simulink model "Detumbling_project"  (R2022b)
settings: Solver=VariableStepAuto  StartTime=0.0  StopTime=400  RelTol=1e-3
values from neighbouring files (symbols this model uses):
  a = (Rp+Ra)/2    [trial_complete_project.m]    (also in trial_detumbling.m; trial_earth_pointing.m)
  A0 = Ax*Ay*Az    [trial_complete_project.m]    (also in trial_detumbling.m = [0.5391 0.1008 0.8362; -0.3591 0.9255 0.1200; -0.7618 -0.365; trial_earth_pointing.m = [-0.2505 -0.7848 0.5668; 0.7978 0.1644 0.5801; -0.5485 0.597)
  A1 = L1*L2    (= 0.06)    [trial_complete_project.m]    (also in trial_detumbling.m; trial_earth_pointing.m)
  A10 = A1    (= 0.06)    [trial_complete_project.m]    (also in trial_detumbling.m; trial_earth_pointing.m)
  A2 = A1    (= 0.06)    [trial_complete_project.m]    (also in trial_detumbling.m; trial_earth_pointing.m)
  A3 = L1*L3    (= 0.03)    [trial_complete_project.m]    (also in trial_detumbling.m; trial_earth_pointing.m)
  A4 = A3    (= 0.03)    [trial_complete_project.m]    (also in trial_detumbling.m; trial_earth_pointing.m)
  A5 = L2*L3    (= 0.02)    [trial_complete_project.m]    (also in trial_detumbling.m; trial_earth_pointing.m)
  A6 = A5    (= 0.02)    [trial_complete_project.m]    (also in trial_detumbling.m; trial_earth_pointing.m)
  A7 = A1    (= 0.06)    [trial_complete_project.m]    (also in trial_detumbling.m; trial_earth_pointing.m)
  A8 = A1    (= 0.06)    [trial_complete_project.m]    (also in trial_detumbling.m; trial_earth_pointing.m)
  A9 = A1    (= 0.06)    [trial_complete_project.m]    (also in trial_detumbling.m; trial_earth_pointing.m)
  a_s = 149600000    [trial_complete_project.m]    (also in trial_detumbling.m; trial_earth_pointing.m)
  alpha1 = 0.9    [trial_complete_project.m]    (also in trial_detumbling.m; trial_earth_pointing.m)
  alpha2 = 0.1    [trial_complete_project.m]    (also in trial_detumbling.m; trial_earth_pointing.m)
  alphaState_obs = -0.9    [trial_complete_project.m]    (also in trial_detumbling.m; trial_earth_pointing.m)
  an = (11.5*pi)/180    (= 0.200712863979)    [trial_complete_project.m]    (also in trial_detumbling.m; trial_earth_pointing.m)
  d = 0.05/2    (= 0.025)    [trial_complete_project.m]    (also in trial_detumbling.m; trial_earth_pointing.m)
  e = (Ra-Rp)/(Ra+Rp)    [trial_complete_project.m]    (also in trial_detumbling.m; trial_earth_pointing.m)
  e_s = 0.0167086    [trial_complete_project.m]    (also in trial_detumbling.m; trial_earth_pointing.m)
  g_vect = g_vect'.*1e-9    [trial_complete_project.m]    (also in trial_detumbling.m; trial_earth_pointing.m)
  gamma = 30*pi/180    (= 0.523598775598)    [trial_complete_project.m]    (also in trial_detumbling.m; trial_earth_pointing.m)
  h_vect = h_vect'.*1e-9    [trial_complete_project.m]    (also in trial_detumbling.m; trial_earth_pointing.m)
  i = 0*pi/180    (= 0)    [trial_complete_project.m]    (also in trial_detumbling.m; trial_earth_pointing.m)
  I_x = 0.059029338    [trial_complete_project.m]    (also in trial_detumbling.m; trial_earth_pointing.m = 0.093296)
  I_y = 0.116709338    [trial_complete_project.m]    (also in trial_detumbling.m; trial_earth_pointing.m = 0.161261916)
  I_z = 0.149968    [trial_complete_project.m]    (also in trial_detumbling.m; trial_earth_pointing.m = 0.160253916)
  kdx = kd*(I_x/I)    (= 1.44987726319)    [trial_complete_project.m]    (also in trial_detumbling.m; trial_earth_pointing.m = 2.6989394073)
  kdy = kd*(I_y/I)    (= 2.86661211697)    [trial_complete_project.m]    (also in trial_detumbling.m; trial_earth_pointing.m = 4.66511040119)
  kdz = kd*(I_z/I)    (= 3.68351061984)    [trial_complete_project.m]    (also in trial_detumbling.m; trial_earth_pointing.m = 4.63595019151)
  kState_obs = 0.9    [trial_complete_project.m]    (also in trial_detumbling.m; trial_earth_pointing.m)
  L = 0.3/2    (= 0.15)    [trial_complete_project.m]    (also in trial_detumbling.m; trial_earth_pointing.m)
  m = [0.01 0.05 0.01]    [trial_complete_project.m]    (also in trial_detumbling.m; trial_earth_pointing.m)
  MIB = 5*1e-3    (= 0.005)    [trial_complete_project.m]    (also in trial_detumbling.m; trial_earth_pointing.m)
  mu = astroConstants(13)    [trial_complete_project.m]    (also in trial_detumbling.m; trial_earth_pointing.m)
  n = sqrt(mu/a^3)    [trial_complete_project.m]    (also in trial_detumbling.m; trial_earth_pointing.m)
  n_B = 13    [trial_complete_project.m]    (also in trial_detumbling.m; trial_earth_pointing.m)
  n_s = sqrt(mu_s/a_s^3)    [trial_complete_project.m]    (also in trial_detumbling.m; trial_earth_pointing.m)
  P = F_e/c    (= 4.52980041279e-06)    [trial_complete_project.m]    (also in trial_detumbling.m; trial_earth_pointing.m)
  P_E = F_earth/c    (= 2.23487943783e-06)    [trial_complete_project.m]    (also in trial_detumbling.m; trial_earth_pointing.m)
  pd_sc = 0.1    [trial_complete_project.m]    (also in trial_detumbling.m; trial_earth_pointing.m)
  pd_sp = 0.1    [trial_complete_project.m]    (also in trial_detumbling.m; trial_earth_pointing.m)
  ps_sc = 0.5    [trial_complete_project.m]    (also in trial_detumbling.m; trial_earth_pointing.m)
  ps_sp = 0.1    [trial_complete_project.m]    (also in trial_detumbling.m; trial_earth_pointing.m)
  r = astroConstants(23)    [trial_complete_project.m]    (also in trial_detumbling.m; trial_earth_pointing.m)
  r1 = [0;0;-L3/2] + c_m    [trial_complete_project.m]    (also in trial_detumbling.m; trial_earth_pointing.m)
  r10 = r9    [trial_complete_project.m]    (also in trial_detumbling.m; trial_earth_pointing.m)
  r2 = [0; 0 ;L3/2] + c_m    [trial_complete_project.m]    (also in trial_detumbling.m; trial_earth_pointing.m)
  r3 = [0; L2/2;0] + c_m    [trial_complete_project.m]    (also in trial_detumbling.m; trial_earth_pointing.m)
  r4 = [0; -L2/2;0] + c_m    [trial_complete_project.m]    (also in trial_detumbling.m; trial_earth_pointing.m)
  r5 = [-L1/2; 0 ;0] + c_m    [trial_complete_project.m]    (also in trial_detumbling.m; trial_earth_pointing.m)
  r6 = [L1/2; 0;0]+ c_m    [trial_complete_project.m]    (also in trial_detumbling.m; trial_earth_pointing.m)
  r7 = [-L1/2; 0 ; L3/2 + L1/2] + c_m    [trial_complete_project.m]    (also in trial_detumbling.m; trial_earth_pointing.m)
  r8 = r7    [trial_complete_project.m]    (also in trial_detumbling.m; trial_earth_pointing.m)
  r9 = [-L1/2; 0 ; -L3/2 - L1/2]    [trial_complete_project.m]    (also in trial_detumbling.m; trial_earth_pointing.m)
  theta0 = 0    [trial_complete_project.m]    (also in trial_detumbling.m; trial_earth_pointing.m)
  Thruster_Power = 0.03    [trial_complete_project.m]    (also in trial_detumbling.m; trial_earth_pointing.m)
  w = [1 1 1 1]'    [trial_complete_project.m]    (also in trial_detumbling.m; trial_earth_pointing.m)
  w0_x = 1    [trial_complete_project.m]    (also in trial_detumbling.m; trial_earth_pointing.m = -0.008328)
  w0_y = 1    [trial_complete_project.m]    (also in trial_detumbling.m; trial_earth_pointing.m = 0.004962)
  w0_z = 1    [trial_complete_project.m]    (also in trial_detumbling.m; trial_earth_pointing.m = -0.0004756)
  w_E = (15.04*pi/180)/3600    (= 7.29159776389e-05)    [trial_complete_project.m]    (also in trial_detumbling.m; trial_earth_pointing.m)
libraries: matrix_library x22, vrlib x6, dspinverses x1
(part 2 of 3)

== system Detumbling_project/Attitude Sensors/Magnetometer/H_0 ==
  Constant : Constant  Value=-29615
  Constant1 : Constant  Value=-1728
  Constant2 : Constant  Value=5186
  Display : Display
  Gain : Gain  Gain=1e-9
  Gain1 : Gain  Gain=1e-9
  Gain2 : Gain  Gain=1e-9
  Square : Math  Operator=square
  Square Root : Sqrt
  Square1 : Math  Operator=square
  Square2 : Math  Operator=square
  Sum : Sum  Inputs=|+++
  Output : Outport
  wires:
  Square1/1 -> Sum/2
  Square/1 -> Sum/1
  Square2/1 -> Sum/3
  Sum/1 -> Square Root/1
  Square Root/1 -> Display/1, Output/1
  Constant/1 -> Gain/1
  Gain/1 -> Square/1
  Constant1/1 -> Gain1/1
  Gain1/1 -> Square1/1
  Constant2/1 -> Gain2/1
  Gain2/1 -> Square2/1

== system Detumbling_project/Attitude Sensors/Magnetometer/Theta_integration ==
  Constant : Constant
  Constant1 : Constant  Value=e
  Constant2 : Constant  Value=e
  Constant3 : Constant
  Constant4 : Constant  Value=3/2
  Cos : Trigonometry  Operator=cos
  Divide : Product  Inputs=*/
  Gain : Gain  Gain=n
  Integrator : Integrator  InitialCondition=theta0
  Product : Product
  Scope : Scope
  Scope1 : Scope
  Square : Math  Operator=square
  Square1 : Math  Operator=square
  Square2 : Math  Operator=pow
  Sum : Sum  Inputs=|++
  Sum1 : Sum  Inputs=|+-
  Output : Outport
  wires:
  Constant1/1 -> Product/1
  Integrator/1 -> Output/1, Scope/1, Cos/1
  Constant3/1 -> Sum1/1
  Cos/1 -> Product/2
  Product/1 -> Sum/1
  Square1/1 -> Sum1/2
  Constant/1 -> Sum/2
  Sum1/1 -> Square2/1
  Constant2/1 -> Square1/1
  Square/1 -> Gain/1
  Divide/1 -> Scope1/1, Integrator/1
  Sum/1 -> Square/1
  Square2/1 -> Divide/2
  Constant4/1 -> Square2/2
  Gain/1 -> Divide/1

== system Detumbling_project/Attitude Sensors/Magnetometer/b_n ==
  Input2 : Inport
  Input : Inport  Port=2
  Input3 : Inport  Port=3
  Constant : Constant  Value=3
  Constant1 : Constant  Value=r
  Demux : Demux  Outputs=3
  Divide : Product  Inputs=*/  RndMeth=Zero  SaturateOnIntegerOverflow=on
  Dot Product : DotProduct  OutDataTypeStr=Inherit: Inherit via internal rule
  Gain : Gain  Gain=3
  Normalize Vector : vrlib/Utilities/Normalize Vector  maxzero=0
  Normalize Vector1 : vrlib/Utilities/Normalize Vector  maxzero=0
  Product : Product
  Product1 : Product
  Product3 : Product
  Square : Math  Operator=pow
  Square Root : Sqrt
  Square1 : Math  Operator=pow
  Square2 : Math  Operator=square
  Square3 : Math  Operator=square
  Square4 : Math  Operator=square
  Sum : Sum  Inputs=|+-
  Sum1 : Sum  Inputs=|+++
  Output : Outport
  wires:
  Input2/1 -> Demux/1, Normalize Vector/1  "position vector"
  Constant1/1 -> Square/1  "earth radius"
  Constant/1 -> Square1/2, Square/2
  Square/1 -> Product/1
  Input/1 -> Product/2  "H0"
  Product/1 -> Product3/2
  Square1/1 -> Divide/2
  Input3/1 -> Dot Product/1, Sum/2  "m"
  Normalize Vector/1 -> Product1/2, Dot Product/2
  Dot Product/1 -> Gain/1
  Gain/1 -> Product1/1
  Product1/1 -> Sum/1
  Divide/1 -> Normalize Vector1/1
  Demux/3 -> Square4/1
  Demux/2 -> Square3/1
  Demux/1 -> Square2/1
  Square4/1 -> Sum1/3
  Square3/1 -> Sum1/2
  Square2/1 -> Sum1/1
  Sum1/1 -> Square Root/1
  Square Root/1 -> Square1/1
  Sum/1 -> Product3/1
  Product3/1 -> Divide/1
  Normalize Vector1/1 -> Output/1

== system Detumbling_project/Attitude Sensors/Magnetometer/m ==
  Clock : Clock
  Constant : Constant  Value=an
  Cos : Trigonometry  Operator=cos
  Cos1 : Trigonometry  Operator=cos
  Gain : Gain  Gain=w_E
  Product : Product
  Product1 : Product
  Sin : Trigonometry
  Sin1 : Trigonometry
  Vector Concatenate : Concatenate  NumInputs=3
  Output : Outport
  wires:
  Constant/1 -> Cos/1, Sin/1
  Clock/1 -> Gain/1
  Gain/1 -> Cos1/1, Sin1/1
  Sin/1 -> Product1/1, Product/1
  Cos1/1 -> Product/2
  Sin1/1 -> Product1/2
  Product/1 -> Vector Concatenate/1
  Product1/1 -> Vector Concatenate/2
  Cos/1 -> Vector Concatenate/3
  Vector Concatenate/1 -> Output/1

== system Detumbling_project/Attitude Sensors/Magnetometer/r_N ==
  Input1 : Inport
  Constant : Constant  Value=i
  Constant2 : Constant
  Constant3 : Constant  Value=e
  Constant4 : Constant
  Constant5 : Constant  Value=e
  Cos : Trigonometry  Operator=cos
  Cos1 : Trigonometry  Operator=cos
  Cos4 : Trigonometry  Operator=cos
  Divide : Product  Inputs=*/  RndMeth=Zero  SaturateOnIntegerOverflow=on
  Gain : Gain  Gain=a
  Normalize Vector : vrlib/Utilities/Normalize Vector  maxzero=0
  Product{,1,4..5} (4 alike) : Product
  Sin : Trigonometry
  Sin1 : Trigonometry
  Square : Math  Operator=square
  Sum : Sum  Inputs=|+-
  Sum1 : Sum  Inputs=|++
  Vector Concatenate : Concatenate  NumInputs=3
  Output : Outport
  wires:
  Input1/1 -> Cos4/1, Cos/1, Sin/1
  Constant/1 -> Sin1/1, Cos1/1
  Cos/1 -> Vector Concatenate/1
  Sin/1 -> Product1/1, Product/1
  Cos1/1 -> Product/2
  Product/1 -> Vector Concatenate/2
  Sin1/1 -> Product1/2
  Product1/1 -> Vector Concatenate/3
  Constant4/1 -> Sum1/1
  Product5/1 -> Normalize Vector/1
  Constant2/1 -> Sum/1
  Cos4/1 -> Product4/2
  Sum1/1 -> Divide/2
  Constant3/1 -> Square/1
  Product4/1 -> Sum1/2
  Square/1 -> Sum/2
  Gain/1 -> Divide/1
  Sum/1 -> Gain/1
  Constant5/1 -> Product4/1
  Divide/1 -> Product5/1
  Vector Concatenate/1 -> Product5/2
  Normalize Vector/1 -> Output/1

== system Detumbling_project/Constant Thruster/If Action Subsystem/If Action Subsystem ==
  Action Port : ActionPort  ActionPortLabel=if(u1 >= Tmin)
  Constant : Constant  Value=Thruster_Power
  Out1 : Outport
  wires:
  Constant/1 -> Out1/1

== system Detumbling_project/Constant Thruster/If Action Subsystem/If Action Subsystem1 ==
  Action Port : ActionPort  ActionPortLabel=else
  Constant : Constant  Value=0
  Out1 : Outport
  wires:
  Constant/1 -> Out1/1

== system Detumbling_project/Constant Thruster/If Action Subsystem1/If Action Subsystem ==
  Action Port : ActionPort  ActionPortLabel=if(u1 <=- Tmin)
  Constant : Constant  Value=-Thruster_Power
  Out1 : Outport
  wires:
  Constant/1 -> Out1/1

== system Detumbling_project/Constant Thruster/If Action Subsystem1/If Action Subsystem1 ==
  Action Port : ActionPort  ActionPortLabel=else
  Constant : Constant  Value=0
  Out1 : Outport
  wires:
  Constant/1 -> Out1/1

== system Detumbling_project/Constant Thruster/If Action Subsystem2/If Action Subsystem ==
  Action Port : ActionPort  ActionPortLabel=if(u1 >= Tmin)
  Constant : Constant  Value=Thruster_Power
  Out1 : Outport
  wires:
  Constant/1 -> Out1/1

== system Detumbling_project/Constant Thruster/If Action Subsystem2/If Action Subsystem1 ==
  Action Port : ActionPort  ActionPortLabel=else
  Constant : Constant  Value=0
  Out1 : Outport
  wires:
  Constant/1 -> Out1/1

== system Detumbling_project/Constant Thruster/If Action Subsystem3/If Action Subsystem ==
  Action Port : ActionPort  ActionPortLabel=if(u1 <=- Tmin)
  Constant : Constant  Value=-Thruster_Power
  Out1 : Outport
  wires:
  Constant/1 -> Out1/1

== system Detumbling_project/Constant Thruster/If Action Subsystem3/If Action Subsystem1 ==
  Action Port : ActionPort  ActionPortLabel=else
  Constant : Constant  Value=0
  Out1 : Outport
  wires:
  Constant/1 -> Out1/1

== system Detumbling_project/Constant Thruster/If Action Subsystem4/If Action Subsystem ==
  Action Port : ActionPort  ActionPortLabel=if(u1 >= Tmin)
  Constant : Constant  Value=Thruster_Power
  Out1 : Outport
  wires:
  Constant/1 -> Out1/1

== system Detumbling_project/Constant Thruster/If Action Subsystem4/If Action Subsystem1 ==
  Action Port : ActionPort  ActionPortLabel=else
  Constant : Constant  Value=0
  Out1 : Outport
  wires:
  Constant/1 -> Out1/1

== system Detumbling_project/Constant Thruster/If Action Subsystem5/If Action Subsystem ==
  Action Port : ActionPort  ActionPortLabel=if(u1 <=- Tmin)
  Constant : Constant  Value=-Thruster_Power
  Out1 : Outport
  wires:
  Constant/1 -> Out1/1

== system Detumbling_project/Constant Thruster/If Action Subsystem5/If Action Subsystem1 ==
  Action Port : ActionPort  ActionPortLabel=else
  Constant : Constant  Value=0
  Out1 : Outport
  wires:
  Constant/1 -> Out1/1

== system Detumbling_project/Constant Thruster/If Action Subsystem6/If Action Subsystem ==
  Action Port : ActionPort  ActionPortLabel=if(u1 >= Tmin)
  Constant : Constant  Value=Thruster_Power
  Out1 : Outport
  wires:
  Constant/1 -> Out1/1

== system Detumbling_project/Constant Thruster/If Action Subsystem6/If Action Subsystem1 ==
  Action Port : ActionPort  ActionPortLabel=else
  Constant : Constant  Value=0
  Out1 : Outport
  wires:
  Constant/1 -> Out1/1

== system Detumbling_project/Constant Thruster/If Action Subsystem7/If Action Subsystem ==
  Action Port : ActionPort  ActionPortLabel=if(u1 <=- Tmin)
  Constant : Constant  Value=-Thruster_Power
  Out1 : Outport
  wires:
  Constant/1 -> Out1/1

== system Detumbling_project/Constant Thruster/If Action Subsystem7/If Action Subsystem1 ==
  Action Port : ActionPort  ActionPortLabel=else
  Constant : Constant  Value=0
  Out1 : Outport
  wires:
  Constant/1 -> Out1/1

== system Detumbling_project/Environment/ERP Torque/Spacecraft Geometry ==
  Constant : Constant
  Gain : Gain  Gain=-1
  Gain1 : Gain  Gain=-1
  Gain2 : Gain  Gain=-1
  Vector Concatenate : Concatenate  NumInputs=3
  Vector Concatenate1 : Concatenate  NumInputs=3
  Vector Concatenate2 : Concatenate  NumInputs=3
  Zero : Constant  Value=0  OutDataTypeStr=Inherit: Inherit via back propagation
  Output : Outport
  Output1 : Outport  Port=2
  Output2 : Outport  Port=3
  Output3 : Outport  Port=4
  Output4 : Outport  Port=5
  Output5 : Outport  Port=6
  Output6 : Outport  Port=7
  Output7 : Outport  Port=8
  Output8 : Outport  Port=9
  Output9 : Outport  Port=10
  wires:
  Gain/1 -> Output5/1, Output7/1, Output9/1
  Gain1/1 -> Output2/1
  Gain2/1 -> Output1/1
  Vector Concatenate2/1 -> Output/1, Gain2/1
  Vector Concatenate/1 -> Gain/1, Output4/1, Output6/1, Output8/1
  Zero/1 -> Vector Concatenate1/1, Vector Concatenate/2, Vector Concatenate/3, Vector Concatenate1/3, Vector Concatenate2/1, Vector Concatenate2/2
  Vector Concatenate1/1 -> Gain1/1, Output3/1
  Constant/1 -> Vector Concatenate1/2, Vector Concatenate/1, Vector Concatenate2/3

== system Detumbling_project/Environment/ERP Torque/Subsystem ==
  Input : Inport
  Input1 : Inport  Port=2
  Constant : Constant
  Constant1 : Constant  Value=ps_sc
  Constant2 : Constant  Value=pd_sc
  Display : Display
  Dot Product : DotProduct  OutDataTypeStr=Inherit: Inherit via internal rule
  Gain : Gain  Gain=-P_E
  Gain1 : Gain  Gain=A1
  Gain2 : Gain  Gain=2
  Gain3 : Gain  Gain=2/3
  Product{,1..3} (4 alike) : Product
  Sum : Sum  Inputs=|+-
  Sum1 : Sum  Inputs=|++
  Sum2 : Sum  Inputs=|++
  Output : Outport
  Output1 : Outport  Port=2
  wires:
  Gain3/1 -> Sum2/2
  Product3/1 -> Sum1/2
  Constant/1 -> Sum/1
  Gain2/1 -> Product2/1
  Input/1 -> Dot Product/1, Product1/2  "r-B"
  Sum2/1 -> Product3/1
  Gain1/1 -> Product/1
  Gain/1 -> Gain1/1
  Dot Product/1 -> Gain/1, Product2/2, Output1/1
  Product/1 -> Output/1, Display/1
  Sum1/1 -> Product/2
  Constant1/1 -> Sum/2, Gain2/1
  Sum/1 -> Product1/1
  Constant2/1 -> Gain3/1
  Product1/1 -> Sum1/1
  Product2/1 -> Sum2/1
  Input1/1 -> Product3/2, Dot Product/2  "N_B"

== system Detumbling_project/Environment/ERP Torque/Subsystem10 ==
  Input : Inport
  Input1 : Inport  Port=2
  Constant : Constant
  Constant1 : Constant  Value=ps_sp
  Constant2 : Constant  Value=pd_sp
  Dot Product : DotProduct  OutDataTypeStr=Inherit: Inherit via internal rule
  Gain : Gain  Gain=-P_E
  Gain1 : Gain  Gain=A10
  Gain2 : Gain  Gain=2
  Gain3 : Gain  Gain=2/3
  Product{,1..3} (4 alike) : Product
  Sum : Sum  Inputs=|+-
  Sum1 : Sum  Inputs=|++
  Sum2 : Sum  Inputs=|++
  Output : Outport
  Output1 : Outport  Port=2
  wires:
  Input1/1 -> Dot Product/2, Product3/2  "N_B"
  Product2/1 -> Sum2/1
  Product1/1 -> Sum1/1
  Constant2/1 -> Gain3/1
  Sum/1 -> Product1/1
  Constant1/1 -> Gain2/1, Sum/2
  Sum1/1 -> Product/2
  Product/1 -> Output/1
  Dot Product/1 -> Output1/1, Product2/2, Gain/1
  Gain/1 -> Gain1/1
  Gain1/1 -> Product/1
  Sum2/1 -> Product3/1
  Input/1 -> Product1/2, Dot Product/1  "S-B"
  Gain2/1 -> Product2/1
  Constant/1 -> Sum/1
  Product3/1 -> Sum1/2
  Gain3/1 -> Sum2/2

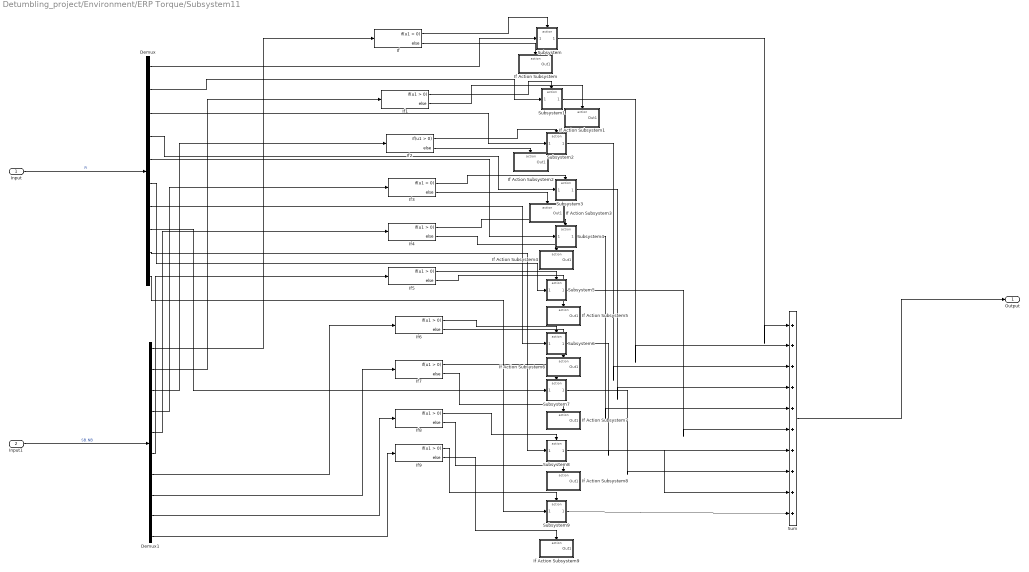
== system Detumbling_project/Environment/ERP Torque/Subsystem11 ==
  Input : Inport
  Input1 : Inport  Port=2
  Demux : Demux  Outputs=10
  Demux1 : Demux  Outputs=10
  If{,1..9} (10 alike) : If  ZeroCross=off
  If Action Subsystem : Subsystem  TreatAsAtomicUnit=on
  If Action Subsystem1 : Subsystem  TreatAsAtomicUnit=on
  If Action Subsystem2 : Subsystem  TreatAsAtomicUnit=on
  If Action Subsystem3 : Subsystem  TreatAsAtomicUnit=on
  If Action Subsystem4 : Subsystem  TreatAsAtomicUnit=on
  If Action Subsystem5 : Subsystem  TreatAsAtomicUnit=on
  If Action Subsystem6 : Subsystem  TreatAsAtomicUnit=on
  If Action Subsystem7 : Subsystem  TreatAsAtomicUnit=on
  If Action Subsystem8 : Subsystem  TreatAsAtomicUnit=on
  If Action Subsystem9 : Subsystem  TreatAsAtomicUnit=on
  Subsystem : Subsystem
  Subsystem1 : Subsystem
  Subsystem2 : Subsystem
  Subsystem3 : Subsystem
  Subsystem4 : Subsystem
  Subsystem5 : Subsystem
  Subsystem6 : Subsystem
  Subsystem7 : Subsystem
  Subsystem8 : Subsystem
  Subsystem9 : Subsystem
  Sum : Sum  Inputs=|++++++++++
  Output : Outport
  wires:
  Sum/1 -> Output/1
  If9/1 -> Subsystem9/Action
  If9/2 -> If Action Subsystem9/Action
  If8/1 -> Subsystem8/Action
  If8/2 -> If Action Subsystem8/Action
  If7/1 -> Subsystem7/Action
  If7/2 -> If Action Subsystem7/Action
  If6/1 -> Subsystem6/Action
  If6/2 -> If Action Subsystem6/Action
  If5/1 -> Subsystem5/Action
  If5/2 -> If Action Subsystem5/Action
  If4/1 -> Subsystem4/Action
  If4/2 -> If Action Subsystem4/Action
  If3/1 -> Subsystem3/Action
  If3/2 -> If Action Subsystem3/Action
  If2/1 -> Subsystem2/Action
  If2/2 -> If Action Subsystem2/Action
  If1/2 -> If Action Subsystem1/Action
  If1/1 -> Subsystem1/Action
  If/2 -> If Action Subsystem/Action
  If/1 -> Subsystem/Action
  Subsystem9/1(Output) -> Sum/10
  Subsystem8/1(Output) -> Sum/9
  Subsystem7/1(Output) -> Sum/8
  Subsystem6/1(Output) -> Sum/7
  Subsystem5/1(Output) -> Sum/6
  Subsystem4/1(Output) -> Sum/5
  Subsystem3/1(Output) -> Sum/4
  Subsystem2/1(Output) -> Sum/3
  Subsystem1/1(Output) -> Sum/2
  Subsystem/1(Output) -> Sum/1
  Demux/10 -> Subsystem9/1(Input3)
  Demux/9 -> Subsystem8/1(Input3)
  Demux/8 -> Subsystem7/1(Input3)
  Demux/7 -> Subsystem6/1(Input3)
  Demux/6 -> Subsystem5/1(Input3)
  Demux/5 -> Subsystem4/1(Input3)
  Demux/4 -> Subsystem3/1(Input3)
  Demux/3 -> Subsystem2/1(Input3)
  Demux/2 -> Subsystem1/1(Input3)
  Demux1/10 -> If9/1
  Demux1/9 -> If8/1
  Demux1/8 -> If7/1
  Demux1/7 -> If6/1
  Demux1/6 -> If5/1
  Demux1/5 -> If4/1
  Demux1/4 -> If3/1
  Demux1/3 -> If2/1
  Demux1/2 -> If1/1
  Demux/1 -> Subsystem/1(Input3)
  Demux1/1 -> If/1
  Input1/1 -> Demux1/1  "SB.NB"
  Input/1 -> Demux/1  "Fi"

== system Detumbling_project/Environment/ERP Torque/Subsystem2 ==
  Input : Inport
  Input1 : Inport  Port=2
  Constant : Constant
  Constant1 : Constant  Value=ps_sc
  Constant2 : Constant  Value=pd_sc
  Dot Product : DotProduct  OutDataTypeStr=Inherit: Inherit via internal rule
  Gain : Gain  Gain=-P_E
  Gain1 : Gain  Gain=A2
  Gain2 : Gain  Gain=2
  Gain3 : Gain  Gain=2/3
  Product{,1..3} (4 alike) : Product
  Sum : Sum  Inputs=|+-
  Sum1 : Sum  Inputs=|++
  Sum2 : Sum  Inputs=|++
  Output : Outport
  Output1 : Outport  Port=2
  wires:
  Input1/1 -> Dot Product/2, Product3/2  "N_B"
  Product2/1 -> Sum2/1
  Product1/1 -> Sum1/1
  Constant2/1 -> Gain3/1
  Sum/1 -> Product1/1
  Constant1/1 -> Gain2/1, Sum/2
  Sum1/1 -> Product/2
  Product/1 -> Output/1
  Dot Product/1 -> Output1/1, Product2/2, Gain/1
  Gain/1 -> Gain1/1
  Gain1/1 -> Product/1
  Sum2/1 -> Product3/1
  Input/1 -> Product1/2, Dot Product/1  "S-B"
  Gain2/1 -> Product2/1
  Constant/1 -> Sum/1
  Product3/1 -> Sum1/2
  Gain3/1 -> Sum2/2

== system Detumbling_project/Environment/ERP Torque/Subsystem3 ==
  Input : Inport
  Input1 : Inport  Port=2
  Constant : Constant
  Constant1 : Constant  Value=ps_sc
  Constant2 : Constant  Value=pd_sc
  Dot Product : DotProduct  OutDataTypeStr=Inherit: Inherit via internal rule
  Gain : Gain  Gain=-P_E
  Gain1 : Gain  Gain=A3
  Gain2 : Gain  Gain=2
  Gain3 : Gain  Gain=2/3
  Product{,1..3} (4 alike) : Product
  Sum : Sum  Inputs=|+-
  Sum1 : Sum  Inputs=|++
  Sum2 : Sum  Inputs=|++
  Output : Outport
  Output1 : Outport  Port=2
  wires:
  Gain3/1 -> Sum2/2
  Product3/1 -> Sum1/2
  Constant/1 -> Sum/1
  Gain2/1 -> Product2/1
  Input/1 -> Dot Product/1, Product1/2  "S-B"
  Sum2/1 -> Product3/1
  Gain1/1 -> Product/1
  Gain/1 -> Gain1/1
  Dot Product/1 -> Gain/1, Product2/2, Output1/1
  Product/1 -> Output/1
  Sum1/1 -> Product/2
  Constant1/1 -> Sum/2, Gain2/1
  Sum/1 -> Product1/1
  Constant2/1 -> Gain3/1
  Product1/1 -> Sum1/1
  Product2/1 -> Sum2/1
  Input1/1 -> Product3/2, Dot Product/2  "N_B"

== system Detumbling_project/Environment/ERP Torque/Subsystem4 ==
  Input : Inport
  Input1 : Inport  Port=2
  Constant : Constant
  Constant1 : Constant  Value=ps_sc
  Constant2 : Constant  Value=pd_sc
  Dot Product : DotProduct  OutDataTypeStr=Inherit: Inherit via internal rule
  Gain : Gain  Gain=-P_E
  Gain1 : Gain  Gain=A4
  Gain2 : Gain  Gain=2
  Gain3 : Gain  Gain=2/3
  Product{,1..3} (4 alike) : Product
  Sum : Sum  Inputs=|+-
  Sum1 : Sum  Inputs=|++
  Sum2 : Sum  Inputs=|++
  Output : Outport
  Output1 : Outport  Port=2
  wires:
  Input1/1 -> Dot Product/2, Product3/2  "N_B"
  Product2/1 -> Sum2/1
  Product1/1 -> Sum1/1
  Constant2/1 -> Gain3/1
  Sum/1 -> Product1/1
  Constant1/1 -> Gain2/1, Sum/2
  Sum1/1 -> Product/2
  Product/1 -> Output/1
  Dot Product/1 -> Output1/1, Product2/2, Gain/1
  Gain/1 -> Gain1/1
  Gain1/1 -> Product/1
  Sum2/1 -> Product3/1
  Input/1 -> Product1/2, Dot Product/1  "S-B"
  Gain2/1 -> Product2/1
  Constant/1 -> Sum/1
  Product3/1 -> Sum1/2
  Gain3/1 -> Sum2/2

== system Detumbling_project/Environment/ERP Torque/Subsystem5 ==
  Input : Inport
  Input1 : Inport  Port=2
  Constant : Constant
  Constant1 : Constant  Value=ps_sc
  Constant2 : Constant  Value=pd_sc
  Dot Product : DotProduct  OutDataTypeStr=Inherit: Inherit via internal rule
  Gain : Gain  Gain=-P_E
  Gain1 : Gain  Gain=A5
  Gain2 : Gain  Gain=2
  Gain3 : Gain  Gain=2/3
  Product{,1..3} (4 alike) : Product
  Sum : Sum  Inputs=|+-
  Sum1 : Sum  Inputs=|++
  Sum2 : Sum  Inputs=|++
  Output : Outport
  Output1 : Outport  Port=2
  wires:
  Gain3/1 -> Sum2/2
  Product3/1 -> Sum1/2
  Constant/1 -> Sum/1
  Gain2/1 -> Product2/1
  Input/1 -> Dot Product/1, Product1/2  "S-B"
  Sum2/1 -> Product3/1
  Gain1/1 -> Product/1
  Gain/1 -> Gain1/1
  Dot Product/1 -> Gain/1, Product2/2, Output1/1
  Product/1 -> Output/1
  Sum1/1 -> Product/2
  Constant1/1 -> Sum/2, Gain2/1
  Sum/1 -> Product1/1
  Constant2/1 -> Gain3/1
  Product1/1 -> Sum1/1
  Product2/1 -> Sum2/1
  Input1/1 -> Product3/2, Dot Product/2  "N_B"

== system Detumbling_project/Environment/ERP Torque/Subsystem6 ==
  Input : Inport
  Input1 : Inport  Port=2
  Constant : Constant
  Constant1 : Constant  Value=ps_sc
  Constant2 : Constant  Value=pd_sc
  Dot Product : DotProduct  OutDataTypeStr=Inherit: Inherit via internal rule
  Gain : Gain  Gain=-P_E
  Gain1 : Gain  Gain=A6
  Gain2 : Gain  Gain=2
  Gain3 : Gain  Gain=2/3
  Product{,1..3} (4 alike) : Product
  Sum : Sum  Inputs=|+-
  Sum1 : Sum  Inputs=|++
  Sum2 : Sum  Inputs=|++
  Output : Outport
  Output1 : Outport  Port=2
  wires:
  Input1/1 -> Dot Product/2, Product3/2  "N_B"
  Product2/1 -> Sum2/1
  Product1/1 -> Sum1/1
  Constant2/1 -> Gain3/1
  Sum/1 -> Product1/1
  Constant1/1 -> Gain2/1, Sum/2
  Sum1/1 -> Product/2
  Product/1 -> Output/1
  Dot Product/1 -> Output1/1, Product2/2, Gain/1
  Gain/1 -> Gain1/1
  Gain1/1 -> Product/1
  Sum2/1 -> Product3/1
  Input/1 -> Product1/2, Dot Product/1  "S-B"
  Gain2/1 -> Product2/1
  Constant/1 -> Sum/1
  Product3/1 -> Sum1/2
  Gain3/1 -> Sum2/2

== system Detumbling_project/Environment/ERP Torque/Subsystem7 ==
  Input : Inport
  Input1 : Inport  Port=2
  Constant : Constant
  Constant1 : Constant  Value=ps_sp
  Constant2 : Constant  Value=pd_sp
  Dot Product : DotProduct  OutDataTypeStr=Inherit: Inherit via internal rule
  Gain : Gain  Gain=-P_E
  Gain1 : Gain  Gain=A7
  Gain2 : Gain  Gain=2
  Gain3 : Gain  Gain=2/3
  Product{,1..3} (4 alike) : Product
  Sum : Sum  Inputs=|+-
  Sum1 : Sum  Inputs=|++
  Sum2 : Sum  Inputs=|++
  Output : Outport
  Output1 : Outport  Port=2
  wires:
  Gain3/1 -> Sum2/2
  Product3/1 -> Sum1/2
  Constant/1 -> Sum/1
  Gain2/1 -> Product2/1
  Input/1 -> Dot Product/1, Product1/2  "S-B"
  Sum2/1 -> Product3/1
  Gain1/1 -> Product/1
  Gain/1 -> Gain1/1
  Dot Product/1 -> Gain/1, Product2/2, Output1/1
  Product/1 -> Output/1
  Sum1/1 -> Product/2
  Constant1/1 -> Sum/2, Gain2/1
  Sum/1 -> Product1/1
  Constant2/1 -> Gain3/1
  Product1/1 -> Sum1/1
  Product2/1 -> Sum2/1
  Input1/1 -> Product3/2, Dot Product/2  "N_B"

== system Detumbling_project/Environment/ERP Torque/Subsystem8 ==
  Input : Inport
  Input1 : Inport  Port=2
  Constant : Constant
  Constant1 : Constant  Value=ps_sp
  Constant2 : Constant  Value=pd_sp
  Dot Product : DotProduct  OutDataTypeStr=Inherit: Inherit via internal rule
  Gain : Gain  Gain=-P_E
  Gain1 : Gain  Gain=A8
  Gain2 : Gain  Gain=2
  Gain3 : Gain  Gain=2/3
  Product{,1..3} (4 alike) : Product
  Sum : Sum  Inputs=|+-
  Sum1 : Sum  Inputs=|++
  Sum2 : Sum  Inputs=|++
  Output : Outport
  Output1 : Outport  Port=2
  wires:
  Input1/1 -> Dot Product/2, Product3/2  "N_B"
  Product2/1 -> Sum2/1
  Product1/1 -> Sum1/1
  Constant2/1 -> Gain3/1
  Sum/1 -> Product1/1
  Constant1/1 -> Gain2/1, Sum/2
  Sum1/1 -> Product/2
  Product/1 -> Output/1
  Dot Product/1 -> Output1/1, Product2/2, Gain/1
  Gain/1 -> Gain1/1
  Gain1/1 -> Product/1
  Sum2/1 -> Product3/1
  Input/1 -> Product1/2, Dot Product/1  "S-B"
  Gain2/1 -> Product2/1
  Constant/1 -> Sum/1
  Product3/1 -> Sum1/2
  Gain3/1 -> Sum2/2

== system Detumbling_project/Environment/ERP Torque/Subsystem9 ==
  Input : Inport
  Input1 : Inport  Port=2
  Constant : Constant
  Constant1 : Constant  Value=ps_sp
  Constant2 : Constant  Value=pd_sp
  Dot Product : DotProduct  OutDataTypeStr=Inherit: Inherit via internal rule
  Gain : Gain  Gain=-P_E
  Gain1 : Gain  Gain=A9
  Gain2 : Gain  Gain=2
  Gain3 : Gain  Gain=2/3
  Product{,1..3} (4 alike) : Product
  Sum : Sum  Inputs=|+-
  Sum1 : Sum  Inputs=|++
  Sum2 : Sum  Inputs=|++
  Output : Outport
  Output1 : Outport  Port=2
  wires:
  Gain3/1 -> Sum2/2
  Product3/1 -> Sum1/2
  Constant/1 -> Sum/1
  Gain2/1 -> Product2/1
  Input/1 -> Dot Product/1, Product1/2  "S-B"
  Sum2/1 -> Product3/1
  Gain1/1 -> Product/1
  Gain/1 -> Gain1/1
  Dot Product/1 -> Gain/1, Product2/2, Output1/1
  Product/1 -> Output/1
  Sum1/1 -> Product/2
  Constant1/1 -> Sum/2, Gain2/1
  Sum/1 -> Product1/1
  Constant2/1 -> Gain3/1
  Product1/1 -> Sum1/1
  Product2/1 -> Sum2/1
  Input1/1 -> Product3/2, Dot Product/2  "N_B"

== system Detumbling_project/Environment/ERP Torque/Theta_integration ==
  Constant : Constant
  Constant1 : Constant  Value=e
  Constant2 : Constant  Value=e
  Constant3 : Constant
  Constant4 : Constant  Value=3/2
  Cos : Trigonometry  Operator=cos
  Divide : Product  Inputs=*/
  Gain : Gain  Gain=n
  Integrator : Integrator  InitialCondition=theta0
  Product : Product
  Scope : Scope
  Square : Math  Operator=square
  Square1 : Math  Operator=square
  Square2 : Math  Operator=pow
  Sum : Sum  Inputs=|++
  Sum1 : Sum  Inputs=|+-
  Output : Outport
  wires:
  Constant1/1 -> Product/1
  Integrator/1 -> Output/1, Scope/1, Cos/1
  Constant3/1 -> Sum1/1
  Cos/1 -> Product/2
  Product/1 -> Sum/1
  Square1/1 -> Sum1/2
  Constant/1 -> Sum/2
  Sum1/1 -> Square2/1
  Constant2/1 -> Square1/1
  Square/1 -> Gain/1
  Divide/1 -> Integrator/1
  Sum/1 -> Square/1
  Square2/1 -> Divide/2
  Constant4/1 -> Square2/2
  Gain/1 -> Divide/1

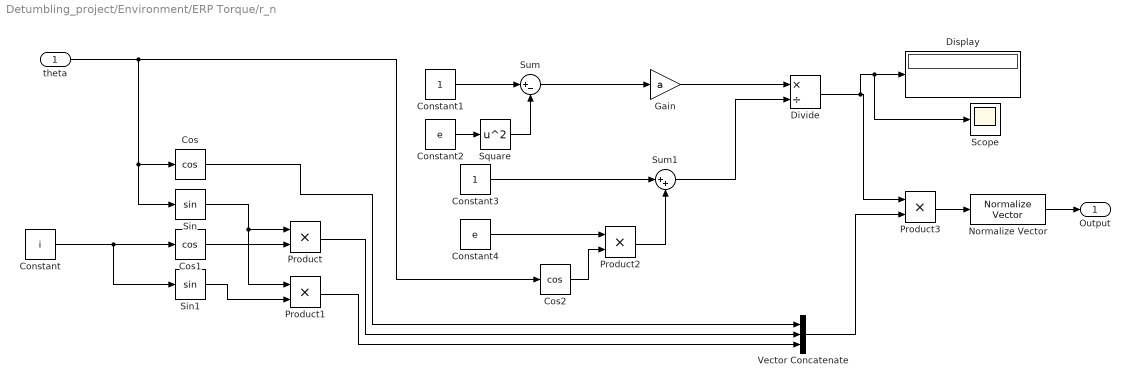
== system Detumbling_project/Environment/ERP Torque/r_n ==
  theta : Inport
  Constant : Constant  Value=i
  Constant1 : Constant
  Constant2 : Constant  Value=e
  Constant3 : Constant
  Constant4 : Constant  Value=e
  Cos : Trigonometry  Operator=cos
  Cos1 : Trigonometry  Operator=cos
  Cos2 : Trigonometry  Operator=cos
  Display : Display
  Divide : Product  Inputs=*/  RndMeth=Zero  SaturateOnIntegerOverflow=on
  Gain : Gain  Gain=a
  Normalize Vector : vrlib/Utilities/Normalize Vector  maxzero=0
  Product{,1..3} (4 alike) : Product
  Scope : Scope
  Sin : Trigonometry
  Sin1 : Trigonometry
  Square : Math  Operator=square
  Sum : Sum  Inputs=|+-
  Sum1 : Sum  Inputs=|++
  Vector Concatenate : Concatenate  NumInputs=3
  Output : Outport
  wires:
  Normalize Vector/1 -> Output/1
  Cos2/1 -> Product2/2
  theta/1 -> Cos/1, Sin/1, Cos2/1
  Vector Concatenate/1 -> Product3/2
  Sin/1 -> Product1/1, Product/1
  Cos/1 -> Vector Concatenate/1
  Product/1 -> Vector Concatenate/2
  Constant/1 -> Sin1/1, Cos1/1
  Sin1/1 -> Product1/2
  Cos1/1 -> Product/2
  Product1/1 -> Vector Concatenate/3
  Constant1/1 -> Sum/1
  Constant2/1 -> Square/1
  Square/1 -> Sum/2
  Sum/1 -> Gain/1
  Gain/1 -> Divide/1
  Constant3/1 -> Sum1/1
  Constant4/1 -> Product2/1
  Product2/1 -> Sum1/2
  Sum1/1 -> Divide/2
  Divide/1 -> Product3/1, Display/1, Scope/1
  Product3/1 -> Normalize Vector/1

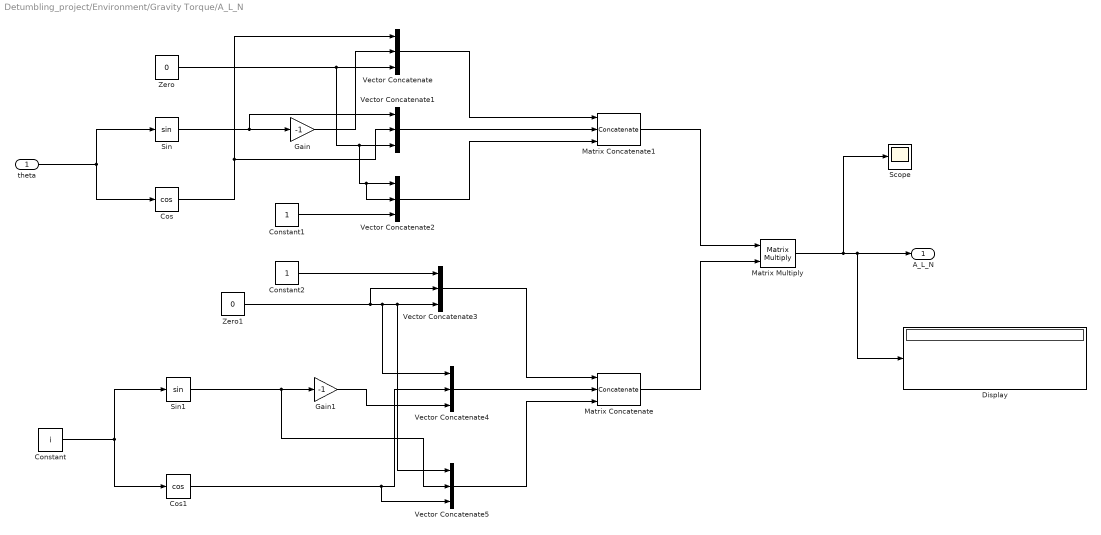
== system Detumbling_project/Environment/Gravity Torque/A_L_N ==
  theta : Inport
  Constant : Constant  Value=i
  Constant1 : Constant
  Constant2 : Constant
  Cos : Trigonometry  Operator=cos
  Cos1 : Trigonometry  Operator=cos
  Display : Display
  Gain : Gain  Gain=-1
  Gain1 : Gain  Gain=-1
  Matrix Concatenate : Concatenate  NumInputs=3  Mode=Multidimensional array  ConcatenateDimension=2
  Matrix Concatenate1 : Concatenate  NumInputs=3  Mode=Multidimensional array  ConcatenateDimension=2
  Matrix Multiply : Product  Multiplication=Matrix(*)
  Scope : Scope
  Sin : Trigonometry
  Sin1 : Trigonometry
  Vector Concatenate{,1..5} (6 alike) : Concatenate  NumInputs=3
  Zero : Constant  Value=0  OutDataTypeStr=Inherit: Inherit via back propagation
  Zero1 : Constant  Value=0  OutDataTypeStr=Inherit: Inherit via back propagation
  A_L_N : Outport
  wires:
  theta/1 -> Sin/1, Cos/1
  Sin/1 -> Vector Concatenate1/1, Gain/1
  Constant/1 -> Cos1/1, Sin1/1
  Sin1/1 -> Vector Concatenate5/2, Gain1/1
  Cos/1 -> Vector Concatenate1/2, Vector Concatenate/1
  Gain/1 -> Vector Concatenate/2
  Zero/1 -> Vector Concatenate2/2, Vector Concatenate2/1, Vector Concatenate1/3, Vector Concatenate/3
  Constant1/1 -> Vector Concatenate2/3
  Constant2/1 -> Vector Concatenate3/1
  Zero1/1 -> Vector Concatenate3/2, Vector Concatenate4/1, Vector Concatenate5/1, Vector Concatenate3/3
  Cos1/1 -> Vector Concatenate5/3, Vector Concatenate4/2
  Gain1/1 -> Vector Concatenate4/3
  Vector Concatenate3/1 -> Matrix Concatenate/1
  Vector Concatenate4/1 -> Matrix Concatenate/2
  Vector Concatenate5/1 -> Matrix Concatenate/3
  Vector Concatenate/1 -> Matrix Concatenate1/1
  Vector Concatenate1/1 -> Matrix Concatenate1/2
  Vector Concatenate2/1 -> Matrix Concatenate1/3
  Matrix Concatenate/1 -> Matrix Multiply/2
  Matrix Concatenate1/1 -> Matrix Multiply/1
  Matrix Multiply/1 -> Scope/1, Display/1, A_L_N/1

== system Detumbling_project/Environment/Gravity Torque/Two_body_problem ==
  R : Subsystem
  Theta_integration : Subsystem
  r : Outport
  theta : Outport  Port=2
  wires:
  Theta_integration/1(Output) -> theta/1, R/1(Input)
  R/1(Output) -> r/1

== system Detumbling_project/Environment/Gravity Torque/grav_torque ==
  Input : Inport
  Input1 : Inport  Port=2
  Constant : Constant  Value=3
  Constant1 : Constant  Value=3*mu
  Demux : Demux  Outputs=3
  Divide : Product  Inputs=*/  RndMeth=Zero  SaturateOnIntegerOverflow=on
  Gain : Gain  Gain=(I_z-I_y)
  Gain1 : Gain  Gain=(I_x-I_z)
  Gain2 : Gain  Gain=(I_y-I_x)
  Mux : Mux  Inputs=3
  Product{,1..5} (6 alike) : Product
  Square : Math  Operator=pow
  Output : Outport
  wires:
  Input/1 -> Demux/1
  Demux/3 -> Product1/2, Product/1
  Demux/2 -> Product2/1, Product/2
  Demux/1 -> Product2/2, Product1/1
  Product/1 -> Gain/1
  Product1/1 -> Gain1/1
  Product2/1 -> Gain2/1
  Mux/1 -> Output/1
  Input1/1 -> Square/1
  Constant1/1 -> Divide/1
  Square/1 -> Divide/2
  Constant/1 -> Square/2
  Gain/1 -> Product3/1
  Gain1/1 -> Product4/1
  Gain2/1 -> Product5/1
  Divide/1 -> Product5/2, Product4/2, Product3/2
  Product3/1 -> Mux/1
  Product4/1 -> Mux/2
  Product5/1 -> Mux/3

== system Detumbling_project/Environment/Magnetic Torque/MAGNETIC FIELD ==
  S/C position : Inport
  Clock : Clock
  Constant1 : Constant  Value=g_vect
  Constant2 : Constant  Value=h_vect
  MATLAB Function1 : MATLAB Function  TreatAsAtomicUnit=on
  MATLAB Function2 : MATLAB Function  TreatAsAtomicUnit=on
  "order n " : Constant  Value=n_B
  B_n : Outport
  wires:
  Constant2/1 -> MATLAB Function1/7(hS)
  Constant1/1 -> MATLAB Function1/6(gS)
  MATLAB Function2/3(lat) -> MATLAB Function1/4(lat)
  MATLAB Function2/4(lon) -> MATLAB Function1/5(lon)
  Clock/1 -> MATLAB Function2/2(t)
  MATLAB Function2/1(r) -> MATLAB Function1/2(r)
  S/C position/1 -> MATLAB Function2/1(R)
  MATLAB Function2/2(alpha) -> MATLAB Function1/3(alpha)
  "order n "/1 -> MATLAB Function1/1(n_B)
  MATLAB Function1/1(B) -> B_n/1  "B_n"

== system Detumbling_project/Environment/Magnetic Torque/Theta_integration ==
  Constant : Constant
  Constant1 : Constant  Value=e
  Constant2 : Constant  Value=e
  Constant3 : Constant
  Constant4 : Constant  Value=3/2
  Cos : Trigonometry  Operator=cos
  Divide : Product  Inputs=*/
  Gain : Gain  Gain=n
  Integrator : Integrator  InitialCondition=theta0
  Product : Product
  Scope : Scope
  Scope1 : Scope
  Square : Math  Operator=square
  Square1 : Math  Operator=square
  Square2 : Math  Operator=pow
  Sum : Sum  Inputs=|++
  Sum1 : Sum  Inputs=|+-
  Output : Outport
  wires:
  Constant1/1 -> Product/1
  Integrator/1 -> Output/1, Scope/1, Cos/1
  Constant3/1 -> Sum1/1
  Cos/1 -> Product/2
  Product/1 -> Sum/1
  Square1/1 -> Sum1/2
  Constant/1 -> Sum/2
  Sum1/1 -> Square2/1
  Constant2/1 -> Square1/1
  Square/1 -> Gain/1
  Divide/1 -> Scope1/1, Integrator/1
  Sum/1 -> Square/1
  Square2/1 -> Divide/2
  Constant4/1 -> Square2/2
  Gain/1 -> Divide/1

== system Detumbling_project/Environment/Magnetic Torque/r_N ==
  Input1 : Inport
  Constant : Constant  Value=i
  Constant2 : Constant
  Constant3 : Constant  Value=e
  Constant4 : Constant
  Constant5 : Constant  Value=e
  Cos : Trigonometry  Operator=cos
  Cos1 : Trigonometry  Operator=cos
  Cos4 : Trigonometry  Operator=cos
  Divide : Product  Inputs=*/  RndMeth=Zero  SaturateOnIntegerOverflow=on
  Gain : Gain  Gain=a
  Product{,1,4..5} (4 alike) : Product
  Sin : Trigonometry
  Sin1 : Trigonometry
  Square : Math  Operator=square
  Sum : Sum  Inputs=|+-
  Sum1 : Sum  Inputs=|++
  Vector Concatenate : Concatenate  NumInputs=3
  Output : Outport
  wires:
  Input1/1 -> Cos4/1, Cos/1, Sin/1
  Constant/1 -> Sin1/1, Cos1/1
  Cos/1 -> Vector Concatenate/1
  Sin/1 -> Product1/1, Product/1
  Cos1/1 -> Product/2
  Product/1 -> Vector Concatenate/2
  Sin1/1 -> Product1/2
  Product1/1 -> Vector Concatenate/3
  Constant4/1 -> Sum1/1
  Product5/1 -> Output/1
  Constant2/1 -> Sum/1
  Cos4/1 -> Product4/2
  Sum1/1 -> Divide/2
  Constant3/1 -> Square/1
  Product4/1 -> Sum1/2
  Square/1 -> Sum/2
  Gain/1 -> Divide/1
  Sum/1 -> Gain/1
  Constant5/1 -> Product4/1
  Divide/1 -> Product5/1
  Vector Concatenate/1 -> Product5/2

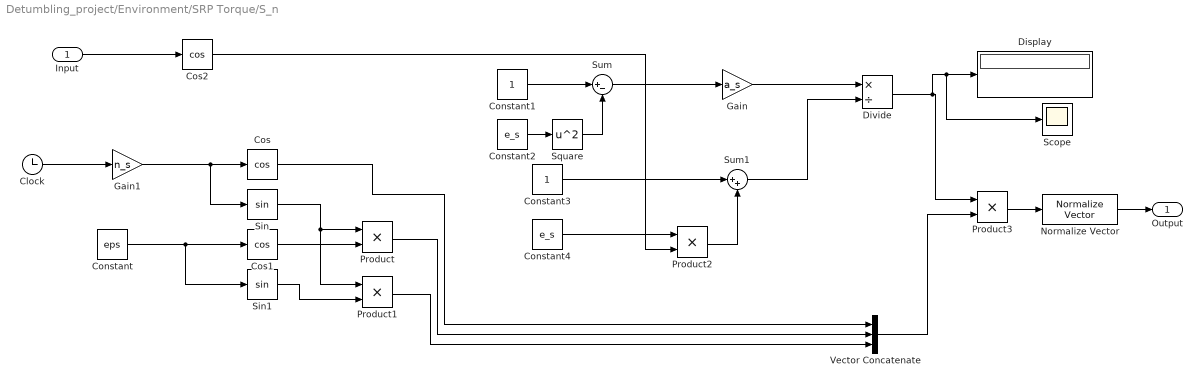
== system Detumbling_project/Environment/SRP Torque/S_n ==
  Input : Inport
  Clock : Clock
  Constant : Constant  Value=eps
  Constant1 : Constant
  Constant2 : Constant  Value=e_s
  Constant3 : Constant
  Constant4 : Constant  Value=e_s
  Cos : Trigonometry  Operator=cos
  Cos1 : Trigonometry  Operator=cos
  Cos2 : Trigonometry  Operator=cos
  Display : Display
  Divide : Product  Inputs=*/  RndMeth=Zero  SaturateOnIntegerOverflow=on
  Gain : Gain  Gain=a_s
  Gain1 : Gain  Gain=n_s
  Normalize Vector : vrlib/Utilities/Normalize Vector  maxzero=0
  Product{,1..3} (4 alike) : Product
  Scope : Scope
  Sin : Trigonometry
  Sin1 : Trigonometry
  Square : Math  Operator=square
  Sum : Sum  Inputs=|+-
  Sum1 : Sum  Inputs=|++
  Vector Concatenate : Concatenate  NumInputs=3
  Output : Outport
  wires:
  Product3/1 -> Normalize Vector/1
  Divide/1 -> Scope/1, Display/1, Product3/1
  Sum1/1 -> Divide/2
  Product2/1 -> Sum1/2
  Constant4/1 -> Product2/1
  Constant3/1 -> Sum1/1
  Gain/1 -> Divide/1
  Sum/1 -> Gain/1
  Square/1 -> Sum/2
  Constant2/1 -> Square/1
  Constant1/1 -> Sum/1
  Product1/1 -> Vector Concatenate/3
  Cos1/1 -> Product/2
  Sin1/1 -> Product1/2
  Constant/1 -> Cos1/1, Sin1/1
  Product/1 -> Vector Concatenate/2
  Cos/1 -> Vector Concatenate/1
  Sin/1 -> Product/1, Product1/1
  Vector Concatenate/1 -> Product3/2
  Clock/1 -> Gain1/1
  Gain1/1 -> Sin/1, Cos/1
  Input/1 -> Cos2/1
  Cos2/1 -> Product2/2
  Normalize Vector/1 -> Output/1

== system Detumbling_project/Environment/SRP Torque/Spacecraft Geometry ==
  Constant : Constant
  Gain : Gain  Gain=-1
  Gain1 : Gain  Gain=-1
  Gain2 : Gain  Gain=-1
  Vector Concatenate : Concatenate  NumInputs=3
  Vector Concatenate1 : Concatenate  NumInputs=3
  Vector Concatenate2 : Concatenate  NumInputs=3
  Zero : Constant  Value=0  OutDataTypeStr=Inherit: Inherit via back propagation
  Output : Outport
  Output1 : Outport  Port=2
  Output2 : Outport  Port=3
  Output3 : Outport  Port=4
  Output4 : Outport  Port=5
  Output5 : Outport  Port=6
  Output6 : Outport  Port=7
  Output7 : Outport  Port=8
  Output8 : Outport  Port=9
  Output9 : Outport  Port=10
  wires:
  Constant/1 -> Vector Concatenate2/3, Vector Concatenate/1, Vector Concatenate1/2
  Vector Concatenate1/1 -> Output3/1, Gain1/1
  Zero/1 -> Vector Concatenate2/2, Vector Concatenate2/1, Vector Concatenate1/3, Vector Concatenate/3, Vector Concatenate/2, Vector Concatenate1/1
  Vector Concatenate/1 -> Output8/1, Output6/1, Output4/1, Gain/1
  Vector Concatenate2/1 -> Gain2/1, Output/1
  Gain2/1 -> Output1/1
  Gain1/1 -> Output2/1
  Gain/1 -> Output9/1, Output7/1, Output5/1

== system Detumbling_project/Environment/SRP Torque/Subsystem ==
  Input : Inport
  Input1 : Inport  Port=2
  Constant : Constant
  Constant1 : Constant  Value=ps_sc
  Constant2 : Constant  Value=pd_sc
  Display : Display
  Dot Product : DotProduct  OutDataTypeStr=Inherit: Inherit via internal rule
  Gain : Gain  Gain=-P
  Gain1 : Gain  Gain=A1
  Gain2 : Gain  Gain=2
  Gain3 : Gain  Gain=2/3
  Product{,1..3} (4 alike) : Product
  Sum : Sum  Inputs=|+-
  Sum1 : Sum  Inputs=|++
  Sum2 : Sum  Inputs=|++
  Output : Outport
  Output1 : Outport  Port=2
  wires:
  Input1/1 -> Dot Product/2, Product3/2  "N_B"
  Product2/1 -> Sum2/1
  Product1/1 -> Sum1/1
  Constant2/1 -> Gain3/1
  Sum/1 -> Product1/1
  Constant1/1 -> Gain2/1, Sum/2
  Sum1/1 -> Product/2
  Product/1 -> Display/1, Output/1
  Dot Product/1 -> Output1/1, Product2/2, Gain/1
  Gain/1 -> Gain1/1
  Gain1/1 -> Product/1
  Sum2/1 -> Product3/1
  Input/1 -> Product1/2, Dot Product/1  "S-B"
  Gain2/1 -> Product2/1
  Constant/1 -> Sum/1
  Product3/1 -> Sum1/2
  Gain3/1 -> Sum2/2

== system Detumbling_project/Environment/SRP Torque/Subsystem10 ==
  Input : Inport
  Input1 : Inport  Port=2
  Constant : Constant
  Constant1 : Constant  Value=ps_sp
  Constant2 : Constant  Value=pd_sp
  Dot Product : DotProduct  OutDataTypeStr=Inherit: Inherit via internal rule
  Gain : Gain  Gain=-P
  Gain1 : Gain  Gain=A10
  Gain2 : Gain  Gain=2
  Gain3 : Gain  Gain=2/3
  Product{,1..3} (4 alike) : Product
  Sum : Sum  Inputs=|+-
  Sum1 : Sum  Inputs=|++
  Sum2 : Sum  Inputs=|++
  Output : Outport
  Output1 : Outport  Port=2
  wires:
  Gain3/1 -> Sum2/2
  Product3/1 -> Sum1/2
  Constant/1 -> Sum/1
  Gain2/1 -> Product2/1
  Input/1 -> Dot Product/1, Product1/2  "S-B"
  Sum2/1 -> Product3/1
  Gain1/1 -> Product/1
  Gain/1 -> Gain1/1
  Dot Product/1 -> Gain/1, Product2/2, Output1/1
  Product/1 -> Output/1
  Sum1/1 -> Product/2
  Constant1/1 -> Sum/2, Gain2/1
  Sum/1 -> Product1/1
  Constant2/1 -> Gain3/1
  Product1/1 -> Sum1/1
  Product2/1 -> Sum2/1
  Input1/1 -> Product3/2, Dot Product/2  "N_B"

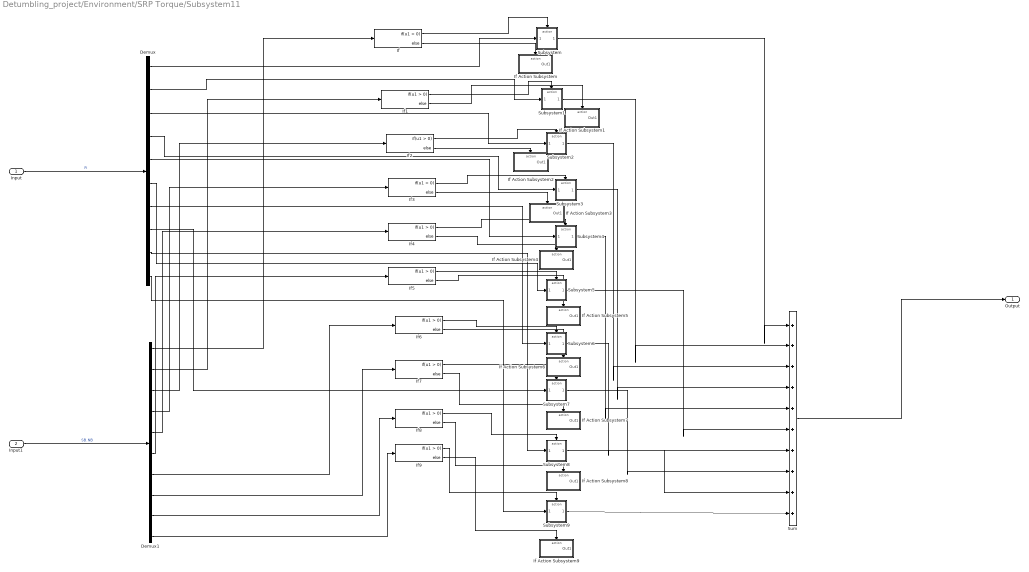
== system Detumbling_project/Environment/SRP Torque/Subsystem11 ==
  Input : Inport
  Input1 : Inport  Port=2
  Demux : Demux  Outputs=10
  Demux1 : Demux  Outputs=10
  If{,1..9} (10 alike) : If  ZeroCross=off
  If Action Subsystem : Subsystem  TreatAsAtomicUnit=on
  If Action Subsystem1 : Subsystem  TreatAsAtomicUnit=on
  If Action Subsystem2 : Subsystem  TreatAsAtomicUnit=on
  If Action Subsystem3 : Subsystem  TreatAsAtomicUnit=on
  If Action Subsystem4 : Subsystem  TreatAsAtomicUnit=on
  If Action Subsystem5 : Subsystem  TreatAsAtomicUnit=on
  If Action Subsystem6 : Subsystem  TreatAsAtomicUnit=on
  If Action Subsystem7 : Subsystem  TreatAsAtomicUnit=on
  If Action Subsystem8 : Subsystem  TreatAsAtomicUnit=on
  If Action Subsystem9 : Subsystem  TreatAsAtomicUnit=on
  Subsystem : Subsystem
  Subsystem1 : Subsystem
  Subsystem2 : Subsystem
  Subsystem3 : Subsystem
  Subsystem4 : Subsystem
  Subsystem5 : Subsystem
  Subsystem6 : Subsystem
  Subsystem7 : Subsystem
  Subsystem8 : Subsystem
  Subsystem9 : Subsystem
  Sum : Sum  Inputs=|++++++++++
  Output : Outport
  wires:
  Input/1 -> Demux/1  "Fi"
  Input1/1 -> Demux1/1  "SB.NB"
  Demux1/1 -> If/1
  Demux/1 -> Subsystem/1(Input3)
  Demux1/2 -> If1/1
  Demux1/3 -> If2/1
  Demux1/4 -> If3/1
  Demux1/5 -> If4/1
  Demux1/6 -> If5/1
  Demux1/7 -> If6/1
  Demux1/8 -> If7/1
  Demux1/9 -> If8/1
  Demux1/10 -> If9/1
  Demux/2 -> Subsystem1/1(Input3)
  Demux/3 -> Subsystem2/1(Input3)
  Demux/4 -> Subsystem3/1(Input3)
  Demux/5 -> Subsystem4/1(Input3)
  Demux/6 -> Subsystem5/1(Input3)
  Demux/7 -> Subsystem6/1(Input3)
  Demux/8 -> Subsystem7/1(Input3)
  Demux/9 -> Subsystem8/1(Input3)
  Demux/10 -> Subsystem9/1(Input3)
  Subsystem/1(Output) -> Sum/1
  Subsystem1/1(Output) -> Sum/2
  Subsystem2/1(Output) -> Sum/3
  Subsystem3/1(Output) -> Sum/4
  Subsystem4/1(Output) -> Sum/5
  Subsystem5/1(Output) -> Sum/6
  Subsystem6/1(Output) -> Sum/7
  Subsystem7/1(Output) -> Sum/8
  Subsystem8/1(Output) -> Sum/9
  Subsystem9/1(Output) -> Sum/10
  If/1 -> Subsystem/Action
  If/2 -> If Action Subsystem/Action
  If1/1 -> Subsystem1/Action
  If1/2 -> If Action Subsystem1/Action
  If2/2 -> If Action Subsystem2/Action
  If2/1 -> Subsystem2/Action
  If3/2 -> If Action Subsystem3/Action
  If3/1 -> Subsystem3/Action
  If4/2 -> If Action Subsystem4/Action
  If4/1 -> Subsystem4/Action
  If5/2 -> If Action Subsystem5/Action
  If5/1 -> Subsystem5/Action
  If6/2 -> If Action Subsystem6/Action
  If6/1 -> Subsystem6/Action
  If7/2 -> If Action Subsystem7/Action
  If7/1 -> Subsystem7/Action
  If8/2 -> If Action Subsystem8/Action
  If8/1 -> Subsystem8/Action
  If9/2 -> If Action Subsystem9/Action
  If9/1 -> Subsystem9/Action
  Sum/1 -> Output/1

== system Detumbling_project/Environment/SRP Torque/Subsystem2 ==
  Input : Inport
  Input1 : Inport  Port=2
  Constant : Constant
  Constant1 : Constant  Value=ps_sc
  Constant2 : Constant  Value=pd_sc
  Dot Product : DotProduct  OutDataTypeStr=Inherit: Inherit via internal rule
  Gain : Gain  Gain=-P
  Gain1 : Gain  Gain=A2
  Gain2 : Gain  Gain=2
  Gain3 : Gain  Gain=2/3
  Product{,1..3} (4 alike) : Product
  Sum : Sum  Inputs=|+-
  Sum1 : Sum  Inputs=|++
  Sum2 : Sum  Inputs=|++
  Output : Outport
  Output1 : Outport  Port=2
  wires:
  Gain3/1 -> Sum2/2
  Product3/1 -> Sum1/2
  Constant/1 -> Sum/1
  Gain2/1 -> Product2/1
  Input/1 -> Dot Product/1, Product1/2  "S-B"
  Sum2/1 -> Product3/1
  Gain1/1 -> Product/1
  Gain/1 -> Gain1/1
  Dot Product/1 -> Gain/1, Product2/2, Output1/1
  Product/1 -> Output/1
  Sum1/1 -> Product/2
  Constant1/1 -> Sum/2, Gain2/1
  Sum/1 -> Product1/1
  Constant2/1 -> Gain3/1
  Product1/1 -> Sum1/1
  Product2/1 -> Sum2/1
  Input1/1 -> Product3/2, Dot Product/2  "N_B"

== system Detumbling_project/Environment/SRP Torque/Subsystem3 ==
  Input : Inport
  Input1 : Inport  Port=2
  Constant : Constant
  Constant1 : Constant  Value=ps_sc
  Constant2 : Constant  Value=pd_sc
  Dot Product : DotProduct  OutDataTypeStr=Inherit: Inherit via internal rule
  Gain : Gain  Gain=-P
  Gain1 : Gain  Gain=A3
  Gain2 : Gain  Gain=2
  Gain3 : Gain  Gain=2/3
  Product{,1..3} (4 alike) : Product
  Sum : Sum  Inputs=|+-
  Sum1 : Sum  Inputs=|++
  Sum2 : Sum  Inputs=|++
  Output : Outport
  Output1 : Outport  Port=2
  wires:
  Input1/1 -> Dot Product/2, Product3/2  "N_B"
  Product2/1 -> Sum2/1
  Product1/1 -> Sum1/1
  Constant2/1 -> Gain3/1
  Sum/1 -> Product1/1
  Constant1/1 -> Gain2/1, Sum/2
  Sum1/1 -> Product/2
  Product/1 -> Output/1
  Dot Product/1 -> Output1/1, Product2/2, Gain/1
  Gain/1 -> Gain1/1
  Gain1/1 -> Product/1
  Sum2/1 -> Product3/1
  Input/1 -> Product1/2, Dot Product/1  "S-B"
  Gain2/1 -> Product2/1
  Constant/1 -> Sum/1
  Product3/1 -> Sum1/2
  Gain3/1 -> Sum2/2

== system Detumbling_project/Environment/SRP Torque/Subsystem4 ==
  Input : Inport
  Input1 : Inport  Port=2
  Constant : Constant
  Constant1 : Constant  Value=ps_sc
  Constant2 : Constant  Value=pd_sc
  Dot Product : DotProduct  OutDataTypeStr=Inherit: Inherit via internal rule
  Gain : Gain  Gain=-P
  Gain1 : Gain  Gain=A4
  Gain2 : Gain  Gain=2
  Gain3 : Gain  Gain=2/3
  Product{,1..3} (4 alike) : Product
  Sum : Sum  Inputs=|+-
  Sum1 : Sum  Inputs=|++
  Sum2 : Sum  Inputs=|++
  Output : Outport
  Output1 : Outport  Port=2
  wires:
  Gain3/1 -> Sum2/2
  Product3/1 -> Sum1/2
  Constant/1 -> Sum/1
  Gain2/1 -> Product2/1
  Input/1 -> Dot Product/1, Product1/2  "S-B"
  Sum2/1 -> Product3/1
  Gain1/1 -> Product/1
  Gain/1 -> Gain1/1
  Dot Product/1 -> Gain/1, Product2/2, Output1/1
  Product/1 -> Output/1
  Sum1/1 -> Product/2
  Constant1/1 -> Sum/2, Gain2/1
  Sum/1 -> Product1/1
  Constant2/1 -> Gain3/1
  Product1/1 -> Sum1/1
  Product2/1 -> Sum2/1
  Input1/1 -> Product3/2, Dot Product/2  "N_B"

== system Detumbling_project/Environment/SRP Torque/Subsystem5 ==
  Input : Inport
  Input1 : Inport  Port=2
  Constant : Constant
  Constant1 : Constant  Value=ps_sc
  Constant2 : Constant  Value=pd_sc
  Dot Product : DotProduct  OutDataTypeStr=Inherit: Inherit via internal rule
  Gain : Gain  Gain=-P
  Gain1 : Gain  Gain=A5
  Gain2 : Gain  Gain=2
  Gain3 : Gain  Gain=2/3
  Product{,1..3} (4 alike) : Product
  Sum : Sum  Inputs=|+-
  Sum1 : Sum  Inputs=|++
  Sum2 : Sum  Inputs=|++
  Output : Outport
  Output1 : Outport  Port=2
  wires:
  Input1/1 -> Dot Product/2, Product3/2  "N_B"
  Product2/1 -> Sum2/1
  Product1/1 -> Sum1/1
  Constant2/1 -> Gain3/1
  Sum/1 -> Product1/1
  Constant1/1 -> Gain2/1, Sum/2
  Sum1/1 -> Product/2
  Product/1 -> Output/1
  Dot Product/1 -> Output1/1, Product2/2, Gain/1
  Gain/1 -> Gain1/1
  Gain1/1 -> Product/1
  Sum2/1 -> Product3/1
  Input/1 -> Product1/2, Dot Product/1  "S-B"
  Gain2/1 -> Product2/1
  Constant/1 -> Sum/1
  Product3/1 -> Sum1/2
  Gain3/1 -> Sum2/2
